simulink model "N3Z_tonetest (conflicted)"  (R2014b)
settings: Solver=ode3  SolverMode=SingleTasking  StartTime=0.0  StopTime=1e-4  FixedStep=fpgaclk  RelTol=1e-3
PreLoadFcn:
  | %fpgaclk=1/32.768e6
  | fpgaclk=1/49.162e6
  | 
  | SerialData=[1,zeros(1,11),1,0,0,1]
  | load ../N3workingG/window
  | win=win';  %Go back to using flatter and wider windowed sync function
  | %load ../N3workingG/hanning    %use Hahn window
  | 
  | load ../N3workingG/PREemphasis   %For pre-empasis and deemphasis FIRs
  | 
  | %LUT3=xls2LUT2('../IQI_Qdemod.xls'); LUT3
  | load ../N3workingG/LUT3
  | load ../N3workingG/FIRiq2
  | % xls2LUT
  | 
  | GetProgFiles
  | 
  | PinAssignments    %Get Pin references for TE0722
  | 
  | 
  | 
  | 
  | 
  | %LCD
  | LCDdata=[LCD_D7,LCD_D6,LCD_D5,LCD_D4,LCD_D3,LCD_D2,LCD_D1,LCD_D0] %Note MSB...LSB!
  | LCDctrl=[LCD_E,LCD_RW,LCD_RS];
  | 
  | %for RS232 on pins 3 and 5 of USBB
  | 
  | %BT chip connections for WT12
  | 
  | RX_BT=RXD
  | TX_BT=TXD
  | 
  | RST_BB=RES
  | 
  | %PCMC=PCMC
  | %PCMS=PCMS
  | %PCMI=PCMI
  | %PCMO=PCMO
  | 
  | %Aliases:
  | SRDBT=PCMI
  | STDBT=PCMO
  | SCLK_BT=PCMC
  | SFS_BT=PCMS
  | 
  | %ADC control
  | 
  | %SDOA=SDOA
  | %SDOB=SDOB
  | %SCK=SCK
  | CONV=Csbar
  | CAL=Cal
  | 
  | ADC_G=[ADC_G3,ADC_G2,ADC_G1,ADC_G0]
  | %PD settings hard coded now
  | 
  | %%%%%%
  | TX_LOW=TX_Low
  | ... (+11 lines)
StartFcn:
  | SerialData=[1,zeros(1,11),1,0,0,1]
values from neighbouring files (symbols this model uses):
  ADC_G0 = {'P10'}    [PinAssignments.m]
  ADC_G1 = {'P11'}    [PinAssignments.m]
  ADC_G2 = {'N14'}    [PinAssignments.m]
  ADC_G3 = {'M11'}    [PinAssignments.m]
  Cal = {'L12'}    [PinAssignments.m]
  Csbar = {'M12'}    [PinAssignments.m]
  LCD_D0 = {'J13'}    [PinAssignments.m]
  LCD_D1 = {'J14'}    [PinAssignments.m]
  LCD_D2 = {'F15'}    [PinAssignments.m]
  LCD_D3 = {'H14'}    [PinAssignments.m]
  LCD_D4 = {'G12'}    [PinAssignments.m]
  LCD_D5 = {'L15'}    [PinAssignments.m]
  LCD_D6 = {'M14'}    [PinAssignments.m]
  LCD_D7 = {'K15'}    [PinAssignments.m]
  PCMC = {'H11'}    [PinAssignments.m]
  PCMI = {'H12'}    [PinAssignments.m]
  PCMO = {'N13'}    [PinAssignments.m]
  PCMS = {'M10'}    [PinAssignments.m]
  RES = {'G11'}    [PinAssignments.m]
  RXD = {'H13'}    [PinAssignments.m]
  TX_Low = {'P15'}    [PinAssignments.m]
  TXD = {'P13'}    [PinAssignments.m]
undefined symbols (not defined in the file or in its folder): AXI4, FIRRX, FIRTX, Lite
libraries: xbsIndex_r4 x1251, MyFunctions x43
(part 3 of 9)

== system N3Z_tonetest (conflicted)/LevelMonitor ==
  note: Add 13-1 (make quicker and reduce level to 7 bits -2014) bits above and below to get ~1.25s time constant
  note: Top 2 bits are sign extended!
  note: Feb 2011 added 1 bit to AddSub unit March 2014, removed 2 bits!
  note: Add lower oscillating bit (but now gives twice the value) - shorter integration
      | but take slice 2 bits lower down - also saturate so as not to wrap around!
  In1 : Inport
  En : Inport  Port=2
  RstPeak : Inport  Port=3
  AddSub : xbsIndex_r4/AddSub  mode=Addition or Subtraction  use_carryin=off  use_carryout=off  en=off  latency=0  precision=User Defined  arith_type=Unsigned  n_bits=22-8+14-1-1  bin_pt=0  quantization=Truncate  overflow=Saturate  use_behavioral_HDL=off  hw_selection=Fabric  pipelined=off  dbl_ovrd=off  block_type=addsub
      settings: block_version=12.2
  AddSub1 : xbsIndex_r4/AddSub  mode=Addition or Subtraction  use_carryin=off  use_carryout=off  en=off  latency=0  precision=User Defined  arith_type=Unsigned  n_bits=8  bin_pt=0  quantization=Truncate  overflow=Saturate  use_behavioral_HDL=off  hw_selection=Fabric  pipelined=off  dbl_ovrd=off  block_type=addsub
      settings: block_version=12.2
  Concat : xbsIndex_r4/Concat  num_inputs=2  dbl_ovrd=off  block_type=concat
      settings: block_version=12.2
  Constant : xbsIndex_r4/Constant  const=0  gui_display_data_type=Fixed-point  arith_type=Signed (2's comp)  n_bits=8  bin_pt=0  preci_type=Single  exp_width=8  frac_width=24  explicit_period=on  period=fpgaclk  equ=P=C  opselect=C  inp2=PCIN>>17  opr=+  inp1=P  carry=CIN  dbl_ovrd=off  block_type=constant
  Convert : xbsIndex_r4/Convert  gui_display_data_type=Boolean  arith_type=Boolean  n_bits=16  bin_pt=14  float_type=Single  exp_bits=8  fraction_bits=24  quantization=Truncate  overflow=Wrap  en=off  latency=0  pipeline=off  dbl_ovrd=off  block_type=convert
      settings: block_version=12.2
  Convert1 : xbsIndex_r4/Convert  gui_display_data_type=Fixed-point  arith_type=Boolean  n_bits=16  bin_pt=14  float_type=Single  exp_bits=8  fraction_bits=24  quantization=Truncate  overflow=Wrap  en=off  latency=0  pipeline=off  dbl_ovrd=off  block_type=convert
      settings: block_version=12.2
  Convert2 : xbsIndex_r4/Convert  gui_display_data_type=Fixed-point  arith_type="Signed  (2's comp)"  n_bits=8  bin_pt=0  float_type=Single  exp_bits=8  fraction_bits=24  quantization=Truncate  overflow=Wrap  en=off  latency=0  pipeline=off  dbl_ovrd=off  block_type=convert
      settings: block_version=12.2
  Counter : xbsIndex_r4/Counter  cnt_type=Free Running  cnt_to=Inf  operation=Up  start_count=0  cnt_by_val=1  arith_type=Unsigned  n_bits=8+13-1  bin_pt=0  load_pin=off  rst=off  en=on  explicit_period=on  period=fpgaclk  use_behavioral_HDL=off  implementation=Fabric  dbl_ovrd=off  block_type=counter
      settings: block_version=12.2
  Counter1 : xbsIndex_r4/Counter  cnt_type=Free Running  cnt_to=Inf  operation=Up  start_count=0  cnt_by_val=1  arith_type=Unsigned  n_bits=1  bin_pt=0  load_pin=off  rst=off  en=on  explicit_period=on  period=fpgaclk  use_behavioral_HDL=off  implementation=Fabric  dbl_ovrd=off  block_type=counter
      settings: block_version=12.2
  Monostable : MyFunctions/Monostable
  Monostable1 : MyFunctions/Monostable
  Register : xbsIndex_r4/Register  init=0  rst=on  en=on  dbl_ovrd=off  block_type=register
      settings: block_version=12.2
  Register1 : xbsIndex_r4/Register  init=0  rst=off  en=on  dbl_ovrd=off  block_type=register
      settings: block_version=12.2
  Register2 : xbsIndex_r4/Register  init=0  rst=on  en=on  dbl_ovrd=off  block_type=register
  Register3 : xbsIndex_r4/Register  init=0  rst=off  en=on  dbl_ovrd=off  block_type=register
      settings: block_version=12.2
  Relational : xbsIndex_r4/Relational  mode=a<b  op_type=Bool  en=off  latency=1  dbl_ovrd=off  block_type=relational
  Slice1 : xbsIndex_r4/Slice  nbits=1  boolean_output=off  mode=Upper Bit Location + Width  bit1=0  base1=MSB of Input  bit0=0  base0=LSB of Input  dbl_ovrd=off  block_type=slice
      settings: block_version=12.2
  Slice2 : xbsIndex_r4/Slice  nbits=1  boolean_output=off  mode=Upper Bit Location + Width  bit1=0  base1=MSB of Input  bit0=0  base0=LSB of Input  dbl_ovrd=off  block_type=slice
      settings: block_version=12.2
  Slice3 : xbsIndex_r4/Slice  nbits=7  boolean_output=off  mode=Upper Bit Location + Width  bit1=0  base1=MSB of Input  bit0=0  base0=LSB of Input  dbl_ovrd=off  block_type=slice
      settings: block_version=12.2
  Slice4 : xbsIndex_r4/Slice  nbits=8  boolean_output=off  mode=Upper Bit Location + Width  bit1=-2  base1=MSB of Input  bit0=0  base0=LSB of Input  dbl_ovrd=off  block_type=slice
      settings: block_version=12.2
  SignalLevel : Outport
  PkSignal : Outport  Port=2
  wires:
  In1/1 -> Slice1/1, Slice4/1
  AddSub/1 -> Register/1
  En/1 -> Register3/2, Register/3, Counter/1
  Slice1/1 -> Convert/1
  Convert/1 -> AddSub1/3, AddSub/3
  Register/1 -> Slice3/1, AddSub/1
  Counter/1 -> Slice2/1
  Monostable/1 -> Convert1/1
  Convert1/1 -> Register/2, Register1/2, Counter1/1
  Slice2/1 -> Monostable/1
  Slice3/1 -> Register1/1
  Slice4/1 -> Convert2/1
  Convert2/1 -> AddSub/2, AddSub1/2
  Register1/1 -> Concat/1
  Counter1/1 -> Concat/2
  Concat/1 -> SignalLevel/1
  Constant/1 -> AddSub1/1
  Register2/1 -> PkSignal/1, Relational/1
  AddSub1/1 -> Register3/1
  Register3/1 -> Relational/2, Register2/1
  Relational/1 -> Monostable1/1
  Monostable1/1 -> Register2/3
  RstPeak/1 -> Register2/2

== system N3Z_tonetest (conflicted)/LevelMonitor1 ==
  In1 : Inport
  En : Inport  Port=2
  RstPeak : Inport  Port=3
  AddSub1 : xbsIndex_r4/AddSub  mode=Addition or Subtraction  use_carryin=off  use_carryout=off  en=off  latency=0  precision=User Defined  arith_type=Unsigned  n_bits=8  bin_pt=0  quantization=Truncate  overflow=Saturate  use_behavioral_HDL=off  hw_selection=Fabric  pipelined=off  dbl_ovrd=off  block_type=addsub
      settings: block_version=12.2
  Constant : xbsIndex_r4/Constant  const=0  gui_display_data_type=Fixed-point  arith_type=Signed (2's comp)  n_bits=8  bin_pt=0  preci_type=Single  exp_width=8  frac_width=24  explicit_period=on  period=fpgaclk  equ=P=C  opselect=C  inp2=PCIN>>17  opr=+  inp1=P  carry=CIN  dbl_ovrd=off  block_type=constant
  Convert : xbsIndex_r4/Convert  gui_display_data_type=Boolean  arith_type=Boolean  n_bits=16  bin_pt=14  float_type=Single  exp_bits=8  fraction_bits=24  quantization=Truncate  overflow=Wrap  en=off  latency=0  pipeline=off  dbl_ovrd=off  block_type=convert
      settings: block_version=12.2
  Convert2 : xbsIndex_r4/Convert  gui_display_data_type=Fixed-point  arith_type="Signed  (2's comp)"  n_bits=8  bin_pt=0  float_type=Single  exp_bits=8  fraction_bits=24  quantization=Truncate  overflow=Wrap  en=off  latency=0  pipeline=off  dbl_ovrd=off  block_type=convert
      settings: block_version=12.2
  Monostable1 : MyFunctions/Monostable
  Register2 : xbsIndex_r4/Register  init=0  rst=on  en=on  dbl_ovrd=off  block_type=register
  Register3 : xbsIndex_r4/Register  init=0  rst=off  en=on  dbl_ovrd=off  block_type=register
      settings: block_version=12.2
  Relational : xbsIndex_r4/Relational  mode=a<b  op_type=Bool  en=off  latency=1  dbl_ovrd=off  block_type=relational
  Slice1 : xbsIndex_r4/Slice  nbits=1  boolean_output=off  mode=Upper Bit Location + Width  bit1=0  base1=MSB of Input  bit0=0  base0=LSB of Input  dbl_ovrd=off  block_type=slice
      settings: block_version=12.2
  Slice4 : xbsIndex_r4/Slice  nbits=8  boolean_output=off  mode=Upper Bit Location + Width  bit1=0  base1=MSB of Input  bit0=0  base0=LSB of Input  dbl_ovrd=off  block_type=slice
      settings: block_version=12.2
  PkSignal : Outport
  wires:
  In1/1 -> Slice1/1, Slice4/1
  En/1 -> Register3/2
  Slice1/1 -> Convert/1
  Convert/1 -> AddSub1/3
  Slice4/1 -> Convert2/1
  Convert2/1 -> AddSub1/2
  Constant/1 -> AddSub1/1
  Register2/1 -> Relational/1, PkSignal/1
  AddSub1/1 -> Register3/1
  Register3/1 -> Register2/1, Relational/2
  Relational/1 -> Monostable1/1
  Monostable1/1 -> Register2/3
  RstPeak/1 -> Register2/2

== system N3Z_tonetest (conflicted)/LoranPulsedetect ==
  Signal : Inport
  Strobe : Inport  Port=2
  FastLevelMonitor : Subsystem
  LoranTrigger : Subsystem
  LranPass : Subsystem
  Trig : Outport
  wires:
  LranPass/1(Out1) -> FastLevelMonitor/1(In1), LoranTrigger/1(LoranSignal)
  FastLevelMonitor/1(SignalLevel) -> LoranTrigger/2(Thresh)
  Signal/1 -> LranPass/1(Signal)
  Strobe/1 -> LranPass/2(Strobe), FastLevelMonitor/2(En)
  LoranTrigger/1(Trig) -> Trig/1

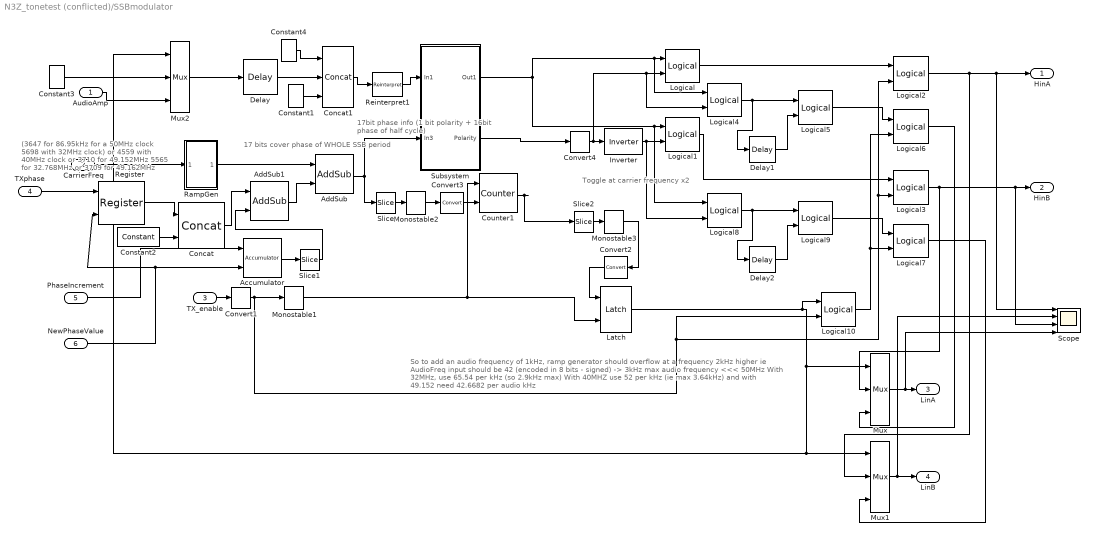
== system N3Z_tonetest (conflicted)/SSBmodulator  ==
  note: (3647 for 86.95kHz for a 50MHz clock
      | 5698 with 32MHz clock)
      | or 4559 with 40MHz clock
      | or 3710 for 49.152MHz
      | 5565 for 32.768MHz
      | or 3709 for 49.162MHz
  note: So to add an audio frequency of 1kHz, ramp generator should overflow at a frequency 2kHz higher
      | ie AudioFreq input should be 42 (encoded in 8 bits - signed) -> 3kHz max audio frequency <<< 50MHz
      | With 32MHz, use 65.54 per kHz (so 2.9kHz max)
      | With 40MHZ use 52 per kHz (ie max 3.64kHz)
      | and with 49.152 need 42.6682 per audio kHz
  note: Toggle at carrier frequency x2
  note: 17bit phase info
      | (1 bit polarity + 16bit phase of half cycle)
  note: 17 bits cover phase of WHOLE SSB period
  AudioAmp : Inport
  CarrierFreq : Inport  Port=2
  TX_enable : Inport  Port=3
  TXphase : Inport  Port=4
  PhaseIncrement : Inport  Port=5
  NewPhaseValue : Inport  Port=6
  Accumulator : xbsIndex_r4/Accumulator  operation=Add  n_bits=19  overflow=Wrap  scale=1  rst=on  hasbypass=off  infoeditControl=reset for floating point data type must be asserted for a minimum of 2 cycles  en=off  latency=0  msb_inp=100  msb=100  lsb=-100  use_behavioral_HDL=on  implementation=Fabric  dbl_ovrd=off  block_type=accum
      settings: block_version=VER_STRING_GOES_HERE
  AddSub : xbsIndex_r4/AddSub  mode=Addition  use_carryin=off  use_carryout=off  en=off  latency=1  precision=User Defined  arith_type=Unsigned  n_bits=17  bin_pt=0  quantization=Truncate  overflow=Wrap  use_behavioral_HDL=off  hw_selection=Fabric  pipelined=off  use_rpm=on  dbl_ovrd=off  block_type=addsub
      settings: block_version=VER_STRING_GOES_HERE
  AddSub1 : xbsIndex_r4/AddSub  mode=Addition  use_carryin=off  use_carryout=off  en=off  latency=0  precision=User Defined  arith_type=Unsigned  n_bits=17  bin_pt=0  quantization=Truncate  overflow=Wrap  use_behavioral_HDL=off  hw_selection=Fabric  pipelined=off  use_rpm=on  dbl_ovrd=off  block_type=addsub
      settings: block_version=VER_STRING_GOES_HERE
  Concat : xbsIndex_r4/Concat  num_inputs=2  dbl_ovrd=off  block_type=concat
      settings: block_version=12.2
  Concat1 : xbsIndex_r4/Concat  num_inputs=3  dbl_ovrd=off  block_type=concat
      settings: block_version=8.2.02
  Constant1 : xbsIndex_r4/Constant  const=0  gui_display_data_type=Fixed-point  arith_type=Unsigned  n_bits=7  bin_pt=0  preci_type=Single  exp_width=8  frac_width=24  explicit_period=on  period=fpgaclk  equ=P=C  opselect=C  inp2=PCIN>>17  opr=+  inp1=P  carry=CIN  dbl_ovrd=off  block_type=constant
      settings: block_version=VER_STRING_GOES_HERE
  Constant2 : xbsIndex_r4/Constant  const=0  gui_display_data_type=Fixed-point  arith_type=Unsigned  n_bits=1  bin_pt=0  preci_type=Single  exp_width=8  frac_width=24  explicit_period=on  period=fpgaclk  equ=P=C  opselect=C  inp2=PCIN>>17  opr=+  inp1=P  carry=CIN  dbl_ovrd=off  block_type=constant
      settings: block_version=12.2
  Constant3 : xbsIndex_r4/Constant  const=40  gui_display_data_type=Fixed-point  arith_type=Unsigned  n_bits=8  bin_pt=0  preci_type=Single  exp_width=8  frac_width=24  explicit_period=on  period=fpgaclk  equ=P=C  opselect=C  inp2=PCIN>>17  opr=+  inp1=P  carry=CIN  dbl_ovrd=off  block_type=constant
      settings: block_version=VER_STRING_GOES_HERE
  Constant4 : xbsIndex_r4/Constant  const=0  gui_display_data_type=Fixed-point  arith_type=Unsigned  n_bits=1  bin_pt=0  preci_type=Single  exp_width=8  frac_width=24  explicit_period=on  period=fpgaclk  equ=P=C  opselect=C  inp2=PCIN>>17  opr=+  inp1=P  carry=CIN  dbl_ovrd=off  block_type=constant
      settings: block_version=VER_STRING_GOES_HERE
  Convert{1..4} (4 alike) : xbsIndex_r4/Convert  gui_display_data_type=Fixed-point  arith_type=Boolean  n_bits=1  bin_pt=0  float_type=Single  exp_bits=8  fraction_bits=24  quantization=Truncate  overflow=Wrap  en=off  latency=0  pipeline=off  dbl_ovrd=off  block_type=convert
      settings: block_version=VER_STRING_GOES_HERE
  Counter1 : xbsIndex_r4/Counter  cnt_type=Free Running  cnt_to=Inf  operation=Up  start_count=0  cnt_by_val=1  arith_type=Unsigned  n_bits=7  bin_pt=0  load_pin=off  rst=on  en=on  explicit_period=off  period=1  use_behavioral_HDL=off  implementation=Fabric  use_rpm=off  dbl_ovrd=off  block_type=counter
      settings: block_version=VER_STRING_GOES_HERE
  Delay : xbsIndex_r4/Delay  rst=off  infoeditControl=Selection of Reset will increase slice count due to use of real FFs and instead of SRLs  en=off  latency=2  reg_retiming=off  dbl_ovrd=off  block_type=delay
      settings: infoedit=Hardware notes: A delay line is a chain, each link of which is an SRL16 followed by a flip-flop. If register retiming is enabled, the delay line is a chain of flip-flops.  block_version=VER_STRING_GOES_HERE
  Delay1 : xbsIndex_r4/Delay  rst=off  infoeditControl=Selection of Reset will increase slice count due to use of real FFs and instead of SRLs  en=off  latency=2  reg_retiming=off  dbl_ovrd=off  block_type=delay
      settings: block_version=12.2
  Delay2 : xbsIndex_r4/Delay  rst=off  infoeditControl=Selection of Reset will increase slice count due to use of real FFs and instead of SRLs  en=off  latency=2  reg_retiming=off  dbl_ovrd=off  block_type=delay
      settings: block_version=12.2
  Inverter : xbsIndex_r4/Inverter  en=off  latency=0  dbl_ovrd=off  block_type=inv
      settings: block_version=VER_STRING_GOES_HERE
  Latch : MyFunctions/Latch
      link override Register2: init=0  rst=on  en=on  dbl_ovrd=off
      link override Set1: arith_type=Boolean  const=1  n_bits=1  bin_pt=0  explicit_period=on  period=fpgaclk  equ=P=C  opselect=C  inp2=PCIN>>17  opr=+  inp1=P  carry=CIN  dbl_ovrd=off  gui_display_data_type=Boolean  preci_type=Single  exp_width=8  frac_width=24
  Logical : xbsIndex_r4/Logical  logical_function=AND  inputs=2  en=off  latency=2  precision=Full  arith_type=Unsigned  n_bits=16  bin_pt=0  align_bp=on  dbl_ovrd=off  block_type=logical
      settings: block_version=VER_STRING_GOES_HERE
  Logical1 : xbsIndex_r4/Logical  logical_function=AND  inputs=2  en=off  latency=2  precision=Full  arith_type=Unsigned  n_bits=16  bin_pt=0  align_bp=on  dbl_ovrd=off  block_type=logical
      settings: block_version=VER_STRING_GOES_HERE
  Logical{2..3,6..7,10} (5 alike) : xbsIndex_r4/Logical  logical_function=AND  inputs=2  en=off  latency=1  precision=Full  arith_type=Unsigned  n_bits=16  bin_pt=0  align_bp=on  dbl_ovrd=off  block_type=logical
      settings: block_version=VER_STRING_GOES_HERE
  Logical4 : xbsIndex_r4/Logical  logical_function=NAND  inputs=2  en=off  latency=1  precision=Full  arith_type=Unsigned  n_bits=16  bin_pt=0  align_bp=on  dbl_ovrd=off  block_type=logical
      settings: block_version=VER_STRING_GOES_HERE
  Logical5 : xbsIndex_r4/Logical  logical_function=AND  inputs=2  en=off  latency=0  precision=Full  arith_type=Unsigned  n_bits=16  bin_pt=0  align_bp=on  dbl_ovrd=off  block_type=logical
      settings: block_version=VER_STRING_GOES_HERE
  Logical8 : xbsIndex_r4/Logical  logical_function=NAND  inputs=2  en=off  latency=1  precision=Full  arith_type=Unsigned  n_bits=16  bin_pt=0  align_bp=on  dbl_ovrd=off  block_type=logical
      settings: block_version=VER_STRING_GOES_HERE
  Logical9 : xbsIndex_r4/Logical  logical_function=AND  inputs=2  en=off  latency=0  precision=Full  arith_type=Unsigned  n_bits=16  bin_pt=0  align_bp=on  dbl_ovrd=off  block_type=logical
      settings: block_version=VER_STRING_GOES_HERE
  Monostable1 : MyFunctions/Monostable
  Monostable2 : MyFunctions/Monostable
  Monostable3 : MyFunctions/Monostable
  Mux : xbsIndex_r4/Mux  inputs=2  en=off  latency=0  precision=Full  arith_type=Unsigned  n_bits=16  bin_pt=14  quantization=Truncate  overflow=Wrap  dbl_ovrd=off  block_type=mux
      settings: block_version=12.2
  Mux1 : xbsIndex_r4/Mux  inputs=2  en=off  latency=0  precision=Full  arith_type=Unsigned  n_bits=16  bin_pt=14  quantization=Truncate  overflow=Wrap  dbl_ovrd=off  block_type=mux
      settings: block_version=12.2
  Mux2 : xbsIndex_r4/Mux  inputs=2  en=off  latency=0  precision=Full  arith_type=Unsigned  n_bits=16  bin_pt=14  quantization=Truncate  overflow=Wrap  dbl_ovrd=off  block_type=mux
      settings: block_version=12.2
  RampGen : Subsystem
  Register : xbsIndex_r4/Register  init=0  rst=off  en=on  dbl_ovrd=off  block_type=register
      settings: block_version=12.2
  Reinterpret1 : xbsIndex_r4/Reinterpret  force_arith_type=on  arith_type=Unsigned  force_bin_pt=on  bin_pt=0  block_type=cast
      settings: infoedit="Changes signal type without altering the binary representation.   You can changed the signal between signed and unsigned, and relocate the binary point.<br><br>Hardware notes: In hardware this block costs nothing.<br><br>Example:  Suppose the input is 6 bits wide, signed, with 2 fractional bits, and the output is forced to unsigned with 0 fractional bits.  Then an input of -2.0 (1110.00 in binary 2's complement) becomes an output of 56 (111000 in binary)."  block_version=VER_STRING_GOES_HERE
  Scope : Scope  NumInputPorts=4
      settings: YMin=-5~-5~-5~-5  YMax=5~5~5~5  MaxDataPoints=50000
  Slice : xbsIndex_r4/Slice  nbits=1  boolean_output=off  mode=Upper Bit Location + Width  bit1=0  base1=MSB of Input  bit0=0  base0=LSB of Input  dbl_ovrd=off  block_type=slice
      settings: block_version=VER_STRING_GOES_HERE
  Slice1 : xbsIndex_r4/Slice  nbits=16  boolean_output=off  mode=Upper Bit Location + Width  bit1=0  base1=MSB of Input  bit0=0  base0=LSB of Input  dbl_ovrd=off  block_type=slice
      settings: block_version=VER_STRING_GOES_HERE
  Slice2 : xbsIndex_r4/Slice  nbits=1  boolean_output=off  mode=Upper Bit Location + Width  bit1=0  base1=MSB of Input  bit0=0  base0=LSB of Input  dbl_ovrd=off  block_type=slice
      settings: block_version=VER_STRING_GOES_HERE
  Subsystem : Subsystem
  HinA : Outport
  HinB : Outport  Port=2
  LinA : Outport  Port=3
  LinB : Outport  Port=4
  wires:
  Subsystem/1(Out1) -> Logical1/1, Logical8/1, Logical/1, Logical4/1
  Reinterpret1/1 -> Subsystem/1(In1)
  Counter1/1 -> Slice2/1
  Slice/1 -> Monostable2/1
  Monostable2/1 -> Convert3/1
  Convert4/1 -> Logical/2, Logical4/2, Inverter/1
  Inverter/1 -> Logical1/2, Logical8/2
  Delay/1 -> Concat1/2
  Concat1/1 -> Reinterpret1/1
  Constant4/1 -> Concat1/1
  Constant1/1 -> Concat1/3
  Logical/1 -> Logical2/1
  Logical1/1 -> Logical3/1
  TX_enable/1 -> Convert1/1
  Logical4/1 -> Logical5/1, Delay1/1
  Delay1/1 -> Logical5/2
  Logical8/1 -> Logical9/1, Delay2/1
  Delay2/1 -> Logical9/2
  Logical5/1 -> Logical6/1
  Logical9/1 -> Logical7/1
  Monostable1/1 -> Latch/2, Counter1/1
  Convert1/1 -> Monostable1/1, Logical10/2, Logical3/2, Logical2/2
  Slice2/1 -> Monostable3/1
  Latch/1 -> Mux/1, Mux1/1, Mux2/1, Logical10/1
  Monostable3/1 -> Convert2/1
  Logical2/1 -> Mux1/2, HinA/1, Scope/1
  Logical3/1 -> Mux/2, HinB/1, Scope/3
  Logical6/1 -> Mux/3
  Logical7/1 -> Mux1/3
  Logical10/1 -> Logical7/2, Logical6/2
  Mux/1 -> LinA/1, Scope/4
  Mux1/1 -> LinB/1, Scope/2
  Convert2/1 -> Latch/1
  Convert3/1 -> Counter1/2
  AudioAmp/1 -> Mux2/3
  Constant3/1 -> Mux2/2
  Mux2/1 -> Delay/1
  RampGen/1(Out1) -> AddSub/1
  AddSub/1 -> Subsystem/2(In3), Slice/1
  CarrierFreq/1 -> RampGen/1(In1)
  Constant2/1 -> Concat/2
  Subsystem/2(Polarity) -> Convert4/1
  Accumulator/1 -> Slice1/1
  Concat/1 -> AddSub1/1
  AddSub1/1 -> AddSub/2
  Slice1/1 -> AddSub1/2
  PhaseIncrement/1 -> Accumulator/1
  NewPhaseValue/1 -> Accumulator/2, Register/2
  TXphase/1 -> Register/1
  Register/1 -> Concat/1

== system N3Z_tonetest (conflicted)/Signed_Unsigned_offset ==
  In1 : Inport
  Concat : xbsIndex_r4/Concat  num_inputs=2  dbl_ovrd=off  block_type=concat
      settings: block_version=VER_STRING_GOES_HERE
  Inverter : xbsIndex_r4/Inverter  en=off  latency=0  dbl_ovrd=off  block_type=inv
      settings: xl_area=[0, 0, 0, 0, 0, 0, 0]  block_version=VER_STRING_GOES_HERE
  Slice2 : xbsIndex_r4/Slice  nbits=13  boolean_output=off  mode=Upper Bit Location + Width  bit1=-1  base1=MSB of Input  bit0=0  base0=LSB of Input  dbl_ovrd=off  block_type=slice
      settings: block_version=VER_STRING_GOES_HERE
  Slice3 : xbsIndex_r4/Slice  nbits=1  boolean_output=off  mode=Upper Bit Location + Width  bit1=0  base1=MSB of Input  bit0=0  base0=LSB of Input  dbl_ovrd=off  block_type=slice
      settings: block_version=VER_STRING_GOES_HERE
  Out1 : Outport
  wires:
  Slice2/1 -> Concat/2
  Slice3/1 -> Inverter/1
  Inverter/1 -> Concat/1
  In1/1 -> Slice2/1, Slice3/1
  Concat/1 -> Out1/1

== system N3Z_tonetest (conflicted)/Subsystem1 ==
  PCMin : Inport
  128kHz : Inport  Port=2
  SFS : Inport  Port=3
  Monostable2 : MyFunctions/Monostable
  Register2 : xbsIndex_r4/Register  init=0  rst=off  en=on  dbl_ovrd=off  block_type=register
      settings: block_version=10.1
  Subsystem1 : Subsystem
  AudioOut : Outport
  wires:
  Register2/1 -> Subsystem1/3(Conv)
  Monostable2/1 -> Register2/2
  PCMin/1 -> Subsystem1/1(SDOA)
  128kHz/1 -> Subsystem1/2(SCK), Monostable2/1
  SFS/1 -> Register2/1
  Subsystem1/1(ADCValueA) -> AudioOut/1

== system N3Z_tonetest (conflicted)/Subsystem2 ==
  note: Counts for 130us
  Signal : Inport
  Strbe : Inport  Port=2
  LoranPulseTrig : Inport  Port=3
  EnableGating : Inport  Port=4
  ADCvalue : xbsIndex_r4/Register  init=0  rst=off  en=on  dbl_ovrd=off  block_type=register
      settings: xl_area=[0, 0, 0, 0, 0, 0, 0]  block_version=VER_STRING_GOES_HERE
  Concat : xbsIndex_r4/Concat  num_inputs=2  dbl_ovrd=off  block_type=concat
      settings: block_version=12.2
  Constant : xbsIndex_r4/Constant  const=9  gui_display_data_type=Fixed-point  arith_type=Unsigned  n_bits=7  bin_pt=0  preci_type=Single  exp_width=8  frac_width=24  explicit_period=on  period=fpgaclk  equ=P=C  opselect=C  inp2=PCIN>>17  opr=+  inp1=P  carry=CIN  dbl_ovrd=off  block_type=constant
      settings: block_version=12.2
  Constant1 : xbsIndex_r4/Constant  const=55  gui_display_data_type=Fixed-point  arith_type=Unsigned  n_bits=7  bin_pt=0  preci_type=Single  exp_width=8  frac_width=24  explicit_period=on  period=fpgaclk  equ=P=C  opselect=C  inp2=PCIN>>17  opr=+  inp1=P  carry=CIN  dbl_ovrd=off  block_type=constant
      settings: block_version=12.2
  Constant2 : xbsIndex_r4/Constant  const=0  gui_display_data_type=Fixed-point  arith_type=Signed (2's comp)  n_bits=16  bin_pt=15  preci_type=Single  exp_width=8  frac_width=24  explicit_period=on  period=fpgaclk  equ=P=C  opselect=C  inp2=PCIN>>17  opr=+  inp1=P  carry=CIN  dbl_ovrd=off  block_type=constant
      settings: block_version=12.2
  Convert : xbsIndex_r4/Convert  gui_display_data_type=Fixed-point  arith_type=Unsigned  n_bits=1  bin_pt=0  float_type=Single  exp_bits=8  fraction_bits=24  quantization=Truncate  overflow=Wrap  en=off  latency=0  pipeline=off  dbl_ovrd=off  block_type=convert
      settings: block_version=12.2
  Convert1 : xbsIndex_r4/Convert  gui_display_data_type=Fixed-point  arith_type=Unsigned  n_bits=1  bin_pt=0  float_type=Single  exp_bits=8  fraction_bits=24  quantization=Truncate  overflow=Wrap  en=off  latency=0  pipeline=off  dbl_ovrd=off  block_type=convert
      settings: block_version=12.2
  Convert2 : xbsIndex_r4/Convert  gui_display_data_type=Fixed-point  arith_type=Boolean  n_bits=1  bin_pt=0  float_type=Single  exp_bits=8  fraction_bits=24  quantization=Truncate  overflow=Wrap  en=off  latency=0  pipeline=off  dbl_ovrd=off  block_type=convert
      settings: block_version=12.2
  Convert3 : xbsIndex_r4/Convert  gui_display_data_type=Fixed-point  arith_type=Boolean  n_bits=1  bin_pt=0  float_type=Single  exp_bits=8  fraction_bits=24  quantization=Truncate  overflow=Wrap  en=off  latency=0  pipeline=off  dbl_ovrd=off  block_type=convert
      settings: block_version=12.2
  Counter1 : xbsIndex_r4/Counter  cnt_type=Free Running  cnt_to=Inf  operation=Up  start_count=0  cnt_by_val=1  arith_type=Unsigned  n_bits=7  bin_pt=0  load_pin=off  rst=on  en=on  explicit_period=on  period=fpgaclk  use_behavioral_HDL=off  implementation=Fabric  dbl_ovrd=off  block_type=counter
      settings: block_version=12.2
  Delay : xbsIndex_r4/Delay  rst=off  infoeditControl=Selection of Reset will increase slice count due to use of real FFs and instead of SRLs  en=on  latency=15  reg_retiming=off  dbl_ovrd=off  block_type=delay
      settings: block_version=12.2
  Divide2 : Subsystem
  Inverter : xbsIndex_r4/Inverter  en=off  latency=0  dbl_ovrd=off  block_type=inv
      settings: block_version=12.2
  Latch : MyFunctions/Latch
      link override Set1: arith_type=Boolean  const=1  n_bits=1  bin_pt=0  explicit_period=on  period=fpgaclk  equ=P=C  opselect=C  inp2=PCIN>>17  opr=+  inp1=P  carry=CIN  dbl_ovrd=off  gui_display_data_type=Boolean  preci_type=Single  exp_width=8  frac_width=24
  Logical : xbsIndex_r4/Logical  logical_function=AND  inputs=2  en=off  latency=0  precision=Full  arith_type=Unsigned  n_bits=16  bin_pt=0  align_bp=on  dbl_ovrd=off  block_type=logical
      settings: block_version=12.2
  Logical1 : xbsIndex_r4/Logical  logical_function=AND  inputs=2  en=off  latency=0  precision=Full  arith_type=Unsigned  n_bits=16  bin_pt=0  align_bp=on  dbl_ovrd=off  block_type=logical
      settings: block_version=12.2
  Monostable : MyFunctions/Monostable
  Monostable1 : MyFunctions/Monostable
  Mux : xbsIndex_r4/Mux  inputs=4  en=off  latency=0  precision=Full  arith_type=Unsigned  n_bits=16  bin_pt=14  quantization=Truncate  overflow=Wrap  dbl_ovrd=off  block_type=mux
      settings: block_version=12.2
  Relational : xbsIndex_r4/Relational  mode=a>b  op_type=Bool  en=off  latency=1  dbl_ovrd=off  block_type=relational
      settings: block_version=12.2
  Relational1 : xbsIndex_r4/Relational  mode=a<=b  op_type=Bool  en=off  latency=1  dbl_ovrd=off  block_type=relational
      settings: block_version=12.2
  Slice : xbsIndex_r4/Slice  nbits=1  boolean_output=off  mode=Upper Bit Location + Width  bit1=0  base1=MSB of Input  bit0=0  base0=LSB of Input  dbl_ovrd=off  block_type=slice
      settings: block_version=12.2
  Archive : Outport
  CleanedUp : Outport  Port=2
  tag scope: LoranTrig=global
  wires:
  Delay/1 -> Archive/1, Mux/2, Divide2/1(In1)
  Signal/1 -> Delay/1
  Strbe/1 -> Delay/2, ADCvalue/2, Counter1/2
  ADCvalue/1 -> CleanedUp/1
  Monostable/1 -> Latch/1, [LoranTrig]
  Latch/1 -> Inverter/1, Convert/1
  Inverter/1 -> Counter1/1
  Counter1/1 -> Slice/1, Relational1/1, Relational/1
  Slice/1 -> Convert2/1
  Mux/1 -> ADCvalue/1
  Constant/1 -> Relational/2
  Constant1/1 -> Relational1/2
  Relational/1 -> Logical/1
  Relational1/1 -> Logical/2
  Logical/1 -> Convert1/1, Monostable1/1
  Convert/1 -> Concat/2
  Convert1/1 -> Concat/1
  Concat/1 -> Mux/1
  Constant2/1 -> Mux/5
  Divide2/1(Out1) -> Mux/3, Mux/4
  Convert2/1 -> Latch/2
  Logical1/1 -> Monostable/1
  LoranPulseTrig/1 -> Logical1/1
  EnableGating/1 -> Convert3/1
  Convert3/1 -> Logical1/2

== system N3Z_tonetest (conflicted)/Subsystem4 ==
  AudioIn : Inport
  Concat : xbsIndex_r4/Concat  num_inputs=2  dbl_ovrd=off  block_type=concat
      settings: block_version=9.2.01
  Convert1 : xbsIndex_r4/Convert  gui_display_data_type=Fixed-point  arith_type=Boolean  n_bits=16  bin_pt=14  float_type=Single  exp_bits=8  fraction_bits=24  quantization=Truncate  overflow=Wrap  en=off  latency=0  pipeline=off  dbl_ovrd=off  block_type=convert
      settings: block_version=9.2.01
  Convert2 : xbsIndex_r4/Convert  gui_display_data_type=Fixed-point  arith_type=Boolean  n_bits=16  bin_pt=14  float_type=Single  exp_bits=8  fraction_bits=24  quantization=Truncate  overflow=Wrap  en=off  latency=0  pipeline=off  dbl_ovrd=off  block_type=convert
      settings: block_version=9.2.01
  Monostable : MyFunctions/Monostable
  Monostable1 : MyFunctions/Monostable
  Mux : xbsIndex_r4/Mux  inputs=2  en=off  latency=0  precision=Full  arith_type=Unsigned  n_bits=16  bin_pt=14  quantization=Truncate  overflow=Wrap  dbl_ovrd=off  block_type=mux
      settings: block_version=9.2.01
  PCMclock : Subsystem
  Register : xbsIndex_r4/Register  init=0  rst=off  en=on  dbl_ovrd=off  block_type=register
      settings: block_version=10.1
  Register1 : xbsIndex_r4/Register  init=0  rst=off  en=on  dbl_ovrd=off  block_type=register
      settings: block_version=10.1
  Reinterpret : xbsIndex_r4/Reinterpret  force_arith_type=on  arith_type=Unsigned  force_bin_pt=on  bin_pt=0  block_type=reinterpret
      settings: block_version=9.2.01
  Slice : xbsIndex_r4/Slice  nbits=15  boolean_output=off  mode=Lower Bit Location + Width  bit1=0  base1=MSB of Input  bit0=0  base0=LSB of Input  dbl_ovrd=off  block_type=slice
      settings: infoedit="Extracts a given range of bits from each input sample and presents it at the output.  The output type is ordinarily unsigned with binary point at zero, but can be Boolean when the slice is one bit wide.<P><P>Hardware notes: In hardware this block costs nothing."  block_version=9.2.01
  Slice2 : xbsIndex_r4/Slice  nbits=1  boolean_output=off  mode=Upper Bit Location + Width  bit1=0  base1=MSB of Input  bit0=0  base0=LSB of Input  dbl_ovrd=off  block_type=slice
      settings: block_version=9.2.01
  PCMout : Outport
  128kHz : Outport  Port=2
  SFS : Outport  Port=3
  wires:
  PCMclock/2(Clk8kHz) -> Convert2/1
  Convert2/1 -> Monostable/1
  Concat/1 -> Mux/2
  Slice2/1 -> Concat/2, PCMout/1
  Slice/1 -> Concat/1
  Register1/1 -> Slice/1, Slice2/1
  Monostable1/1 -> Register1/2
  Mux/1 -> Register1/1
  Convert1/1 -> Monostable1/1, 128kHz/1
  PCMclock/1(128kHz) -> Convert1/1
  Register/1 -> Mux/3
  Monostable/1 -> Register/2, Mux/1
  AudioIn/1 -> Reinterpret/1
  PCMclock/3(STFS) -> SFS/1
  Reinterpret/1 -> Register/1

== system N3Z_tonetest (conflicted)/ToneDetect ==
  Assert4 : xbsIndex_r4/Assert  assert_type=off  type_source=Explicitly  gui_display_data_type=Fixed-point  arith_type="Signed  (2's comp)"  n_bits=16  bin_pt=14  preci_type=Single  exp_width=8  frac_width=24  assert_rate=on  rate_source=Explicitly  period=fpgaclk  output_port=on  block_type=assert
  Concat : xbsIndex_r4/Concat  num_inputs=4  dbl_ovrd=off  block_type=concat
      settings: block_version=9.2.01
  Constant1 : xbsIndex_r4/Constant  const=0  gui_display_data_type=Fixed-point  arith_type=Unsigned  n_bits=5  bin_pt=0  preci_type=Single  exp_width=8  frac_width=24  explicit_period=on  period=fpgaclk  equ=P=C  opselect=C  inp2=PCIN>>17  opr=+  inp1=P  carry=CIN  dbl_ovrd=off  block_type=constant
  Constant2 : xbsIndex_r4/Constant  const=0  gui_display_data_type=Fixed-point  arith_type=Unsigned  n_bits=8  bin_pt=0  preci_type=Single  exp_width=8  frac_width=24  explicit_period=on  period=fpgaclk  equ=P=C  opselect=C  inp2=PCIN>>17  opr=+  inp1=P  carry=CIN  dbl_ovrd=off  block_type=constant
  Constant4 : xbsIndex_r4/Constant  const=0  gui_display_data_type=Boolean  arith_type=Boolean  n_bits=1  bin_pt=0  preci_type=Single  exp_width=8  frac_width=24  explicit_period=on  period=fpgaclk  equ=P=C  opselect=C  inp2=PCIN>>17  opr=+  inp1=P  carry=CIN  dbl_ovrd=off  block_type=constant
      settings: block_version=VER_STRING_GOES_HERE
  Convert1 : xbsIndex_r4/Convert  gui_display_data_type=Fixed-point  arith_type=Boolean  n_bits=16  bin_pt=0  float_type=Single  exp_bits=8  fraction_bits=24  quantization=Truncate  overflow=Wrap  en=off  latency=0  pipeline=off  dbl_ovrd=off  block_type=convert
      settings: xl_area=[0 0 0 0 0 0 0]  block_version=VER_STRING_GOES_HERE
  Convert3 : xbsIndex_r4/Convert  gui_display_data_type=Fixed-point  arith_type=Boolean  n_bits=16  bin_pt=0  float_type=Single  exp_bits=8  fraction_bits=24  quantization=Truncate  overflow=Wrap  en=off  latency=0  pipeline=off  dbl_ovrd=off  block_type=convert
      settings: xl_area=[0 0 0 0 0 0 0]  block_version=VER_STRING_GOES_HERE
  Delay : xbsIndex_r4/Delay  rst=off  infoeditControl=Selection of Reset will increase slice count due to use of real FFs and instead of SRLs  en=off  latency=5  reg_retiming=off  dbl_ovrd=off  block_type=delay
      settings: infoedit=Hardware notes: A delay line is a chain, each link of which is an SRL16 or SRL32 followed by a flip-flop.
  Mult : xbsIndex_r4/Mult  precision=Full  arith_type="Signed  (2's comp)"  n_bits=16  bin_pt=14  quantization=Truncate  overflow=Wrap  en=off  latency=3  use_behavioral_HDL=off  opt=Speed  use_embedded=on  optimum_pipeline=off  pipeline=on  dbl_ovrd=off  use_rpm=on  placement_style=Triangular  block_type=mult
  Mux : xbsIndex_r4/Mux  inputs=8  en=off  latency=1  precision=Full  arith_type=Unsigned  n_bits=16  bin_pt=14  quantization=Truncate  overflow=Wrap  dbl_ovrd=off  block_type=mux
      settings: xl_area=[16 0 0 32 0 0 0]  block_version=VER_STRING_GOES_HERE
  OutputRegister : Subsystem
  PicoBlaze6 : xbsIndex_r4/Black Box  init_code=kcpsm6_CE_256_4k_config  sim_method=Inactive  verbose=off  block_type=blackbox2
  ROM : xbsIndex_r4/ROM  depth=256  initVector=(2^15-1)*sin(pi*(0:255)/128)  distributed_mem=Block RAM  rst=off  init_reg=0  en=off  latency=1  gui_display_data_type=Fixed-point  arith_type="Signed  (2's comp)"  n_bits=16  bin_pt=0  preci_type=Single  exp_width=8  frac_width=24  optimize=Area  use_rpm=on  dbl_ovrd=off  block_type=sprom
  Register : xbsIndex_r4/Register  init=0  rst=off  en=on  dbl_ovrd=off  block_type=register
  Slice : xbsIndex_r4/Slice  nbits=8  boolean_output=off  mode=Lower Bit Location + Width  bit1=0  base1=MSB of Input  bit0=0  base0=LSB of Input  dbl_ovrd=off  block_type=slice
      settings: block_version=8.2.02
  Slice1 : xbsIndex_r4/Slice  nbits=8  boolean_output=off  mode=Lower Bit Location + Width  bit1=0  base1=MSB of Input  bit0=8  base0=LSB of Input  dbl_ovrd=off  block_type=slice
      settings: block_version=8.2.02
  Slice2 : xbsIndex_r4/Slice  nbits=3  boolean_output=off  mode=Lower Bit Location + Width  bit1=0  base1=MSB of Input  bit0=0  base0=LSB of Input  dbl_ovrd=off  block_type=slice
      settings: block_version=VER_STRING_GOES_HERE
  Slice3 : xbsIndex_r4/Slice  nbits=8  boolean_output=off  mode=Upper Bit Location + Width  bit1=-8  base1=MSB of Input  bit0=0  base0=LSB of Input  dbl_ovrd=off  block_type=slice
      settings: block_version=8.2.02
  Slice4 : xbsIndex_r4/Slice  nbits=8  boolean_output=off  mode=Upper Bit Location + Width  bit1=0  base1=MSB of Input  bit0=8  base0=LSB of Input  dbl_ovrd=off  block_type=slice
      settings: block_version=8.2.02
  Slice5 : xbsIndex_r4/Slice  nbits=1  boolean_output=off  mode=Lower Bit Location + Width  bit1=0  base1=MSB of Input  bit0=0  base0=LSB of Input  dbl_ovrd=off  block_type=slice
      settings: block_version=VER_STRING_GOES_HERE
  Slice9 : xbsIndex_r4/Slice  nbits=11  boolean_output=off  mode=Lower Bit Location + Width  bit1=0  base1=MSB of Input  bit0=0  base0=LSB of Input  dbl_ovrd=off  block_type=slice
      settings: block_version=VER_STRING_GOES_HERE
  TDPicoAddress : xbsIndex_r4/Gateway Out  inherit_from_input=off  hdl_port=on  rows=1  columns=1  UseAsDAC=off  DACChannel='1'  interface=None  automatic_assignment=on  address_offset=hex2dec('00')  intf_name=''  intf_description=''  timing_constraint=None  locs_specified=off  LOCs={}  io_standard={}  block_type=gatewayout
  TDPicoInstruction : xbsIndex_r4/Gateway In  gui_display_data_type=Fixed-point  arith_type=Unsigned  n_bits=18  bin_pt=0  preci_type=Single  exp_width=8  frac_width=24  rows=1  columns=1  quantization="Round  (unbiased: +/- Inf)"  overflow=Saturate  period=fpgaclk  UseAsADC=off  ADCChannel='1'  interface=None  automatic_assignment=on  address_offset=hex2dec('00')  intf_name=''  intf_description=''  default_value=0  timing_constraint=None  locs_specified=off  LOCs={}  io_standard={}  inherit_from_input=off  hdl_port=on  dbl_ovrd=off  block_type=gatewayin
  TD_portID : xbsIndex_r4/Gateway Out  inherit_from_input=off  hdl_port=on  rows=1  columns=1  UseAsDAC=off  DACChannel='1'  interface=None  automatic_assignment=on  address_offset=hex2dec('00')  intf_name=''  intf_description=''  timing_constraint=None  locs_specified=off  LOCs={}  io_standard={'LVCMOS33'}  block_type=gatewayout
      settings: block_version=VER_STRING_GOES_HERE
  tag scope: NewTDcmd2user=global, SpeakerOn=global, StartToneAmp=global, TDcmd2user=global
  wires:
  PicoBlaze6/4 -> Slice2/1, OutputRegister/2(PortId), TD_portID/1
  PicoBlaze6/3 -> OutputRegister/1(Data)
  Mux/1 -> PicoBlaze6/2
  Constant4/1 -> Convert1/1
  Slice2/1 -> Assert4/1
  Convert1/1 -> PicoBlaze6/3, PicoBlaze6/4
  OutputRegister/1(Cmd2User) -> [TDcmd2user]
  OutputRegister/2(NewCmd) -> [NewTDcmd2user]
  Convert3/1 -> OutputRegister/3(Write)
  Assert4/1 -> Mux/1
  PicoBlaze6/1 -> Slice9/1
  PicoBlaze6/5 -> Convert3/1
  Slice/1 -> Mux/3
  Slice1/1 -> Mux/2
  [FilterredSignal] -> Slice/1, Slice1/1
  Constant1/1 -> Concat/1
  [Strobe] -> Concat/4
  Concat/1 -> Mux/4
  Slice3/1 -> Mux/6
  Slice4/1 -> Mux/5
  Constant2/1 -> Mux/9, Mux/7, Mux/8
  OutputRegister/3(LOMSB) -> ROM/1
  Mult/1 -> Register/1
  Register/1 -> Slice3/1, Slice4/1  "PrevousDemodValue"
  OutputRegister/4(DoDemod) -> Delay/1
  Slice9/1 -> TDPicoAddress/1
  TDPicoInstruction/1 -> PicoBlaze6/1
  [RstPicos] -> PicoBlaze6/5
  Delay/1 -> Register/2
  [FilterredSignal] -> Mult/1
  ROM/1 -> Mult/2
  OutputRegister/6(State) -> Slice5/1
  Slice5/1 -> [SpeakerOn]
  [TX_High] -> Concat/3
  OutputRegister/5(StartToneAmp) -> [StartToneAmp]
  [ToneDetectOff] -> Concat/2

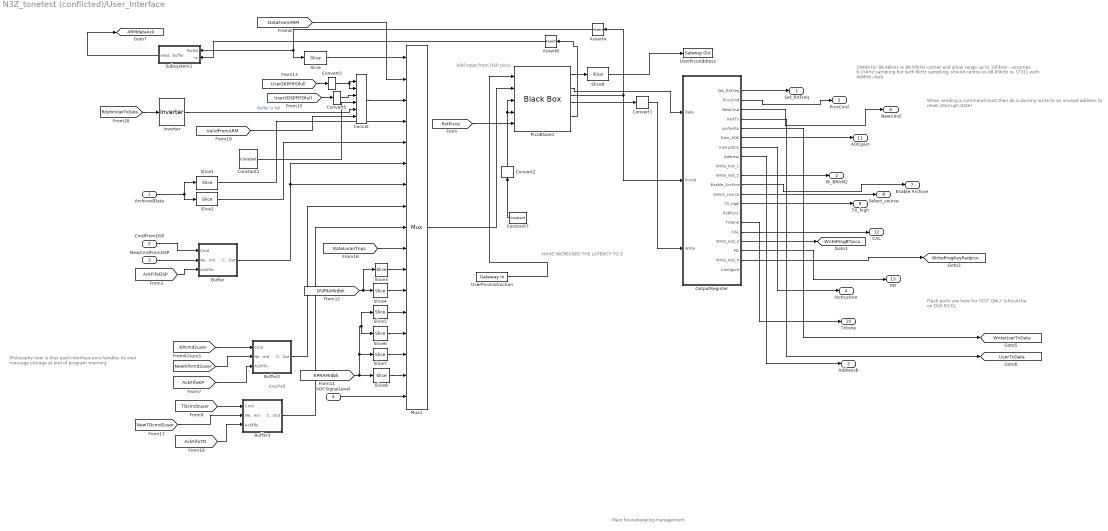
== system N3Z_tonetest (conflicted)/User_Interface ==
  note: When sending a command must then do a dummy write to an unused address
      | to reset interrupt state!
  note: 29689 for 88.48kHz
      |  ie 86.95kHz carrier and allow range up to 195kHz - assumes 6.15kHz sampling
      | but with 8kHz sampling, should centre on 88.95kHz ie 37311 with 40MHz clock
  note: Add input from DSP pico!
  note: Philosophy now is that each interface pico handles its own
      | message storage at end of program memory
  note: Main housekeeping management
  note: KeyPad
  note: Flash ports are here for TEST ONLY (should
      | be on DSP PICO)
  note: HAVE INCREASED THE LATENCY TO 2
  ArchivedData : Inport
  CmdFromDSP : Inport  Port=2
  NewCmdFromDSP : Inport  Port=3
  ADCSignalLevel : Inport  Port=4
  Assert4 : xbsIndex_r4/Assert  assert_type=off  type_source=Explicitly  gui_display_data_type=Fixed-point  arith_type="Signed  (2's comp)"  n_bits=16  bin_pt=14  preci_type=Single  exp_width=8  frac_width=24  assert_rate=on  rate_source=Explicitly  period=fpgaclk  output_port=on  block_type=assert
  Assert6 : xbsIndex_r4/Assert  assert_type=off  type_source=Explicitly  gui_display_data_type=Fixed-point  arith_type="Signed  (2's comp)"  n_bits=16  bin_pt=14  preci_type=Single  exp_width=8  frac_width=24  assert_rate=on  rate_source=Explicitly  period=fpgaclk  output_port=on  block_type=assert
  Buffer : Subsystem
  Buffer2 : Subsystem
  Buffer3 : Subsystem
  Concat : xbsIndex_r4/Concat  num_inputs=6  dbl_ovrd=off  block_type=concat
      settings: block_version=VER_STRING_GOES_HERE
  Constant1 : xbsIndex_r4/Constant  const=0  gui_display_data_type=Fixed-point  arith_type=Unsigned  n_bits=3  bin_pt=0  preci_type=Single  exp_width=8  frac_width=24  explicit_period=on  period=fpgaclk  equ=P=C  opselect=C  inp2=PCIN>>17  opr=+  inp1=P  carry=CIN  dbl_ovrd=off  block_type=constant
      settings: block_version=VER_STRING_GOES_HERE
  Constant7 : xbsIndex_r4/Constant  const=0  gui_display_data_type=Boolean  arith_type=Boolean  n_bits=1  bin_pt=0  preci_type=Single  exp_width=8  frac_width=24  explicit_period=on  period=fpgaclk  equ=P=C  opselect=C  inp2=PCIN>>17  opr=+  inp1=P  carry=CIN  dbl_ovrd=off  block_type=constant
      settings: block_version=VER_STRING_GOES_HERE
  Convert1 : xbsIndex_r4/Convert  gui_display_data_type=Fixed-point  arith_type=Boolean  n_bits=16  bin_pt=0  float_type=Single  exp_bits=8  fraction_bits=24  quantization=Truncate  overflow=Wrap  en=off  latency=0  pipeline=off  dbl_ovrd=off  block_type=convert
      settings: xl_area=[0 0 0 0 0 0 0]  block_version=VER_STRING_GOES_HERE
  Convert2 : xbsIndex_r4/Convert  gui_display_data_type=Fixed-point  arith_type=Boolean  n_bits=16  bin_pt=0  float_type=Single  exp_bits=8  fraction_bits=24  quantization=Truncate  overflow=Wrap  en=off  latency=0  pipeline=off  dbl_ovrd=off  block_type=convert
      settings: xl_area=[0, 0, 0, 0, 0, 0, 0]  block_version=VER_STRING_GOES_HERE
  Convert3 : xbsIndex_r4/Convert  gui_display_data_type=Fixed-point  arith_type=Unsigned  n_bits=1  bin_pt=0  float_type=Single  exp_bits=8  fraction_bits=24  quantization=Truncate  overflow=Wrap  en=off  latency=0  pipeline=off  dbl_ovrd=off  block_type=convert
      settings: xl_area=[0, 0, 0, 0, 0, 0, 0]  block_version=VER_STRING_GOES_HERE
  Convert5 : xbsIndex_r4/Convert  gui_display_data_type=Fixed-point  arith_type=Unsigned  n_bits=1  bin_pt=0  float_type=Single  exp_bits=8  fraction_bits=24  quantization=Truncate  overflow=Wrap  en=off  latency=0  pipeline=off  dbl_ovrd=off  block_type=convert
      settings: xl_area=[0, 0, 0, 0, 0, 0, 0]  block_version=VER_STRING_GOES_HERE
  Inverter : xbsIndex_r4/Inverter  en=off  latency=1  dbl_ovrd=off  block_type=inv
  Mux1 : xbsIndex_r4/Mux  inputs=16  en=off  latency=1  precision=Full  arith_type=Unsigned  n_bits=16  bin_pt=14  quantization=Truncate  overflow=Wrap  dbl_ovrd=off  block_type=mux
      settings: block_version=12.2
  OutputRegister : Subsystem
  PicoBlaze1 : xbsIndex_r4/Black Box  init_code=kcpsm6_CE_256_4k_config  sim_method=Inactive  verbose=off  block_type=blackbox2
  Slice : xbsIndex_r4/Slice  nbits=4  boolean_output=off  mode=Lower Bit Location + Width  bit1=0  base1=MSB of Input  bit0=0  base0=LSB of Input  dbl_ovrd=off  block_type=slice
      settings: block_version=VER_STRING_GOES_HERE
  Slice{1,4,6,8} (4 alike) : xbsIndex_r4/Slice  nbits=8  boolean_output=off  mode=Lower Bit Location + Width  bit1=0  base1=MSB of Input  bit0=0  base0=LSB of Input  dbl_ovrd=off  block_type=slice
      settings: block_version=VER_STRING_GOES_HERE
  Slice{2..3,5,7} (4 alike) : xbsIndex_r4/Slice  nbits=8  boolean_output=off  mode=Lower Bit Location + Width  bit1=0  base1=MSB of Input  bit0=8  base0=LSB of Input  dbl_ovrd=off  block_type=slice
      settings: block_version=VER_STRING_GOES_HERE
  Slice9 : xbsIndex_r4/Slice  nbits=11  boolean_output=off  mode=Lower Bit Location + Width  bit1=0  base1=MSB of Input  bit0=0  base0=LSB of Input  dbl_ovrd=off  block_type=slice
      settings: block_version=VER_STRING_GOES_HERE
  Subsystem1 : Subsystem
  UserPicoAddress : xbsIndex_r4/Gateway Out  inherit_from_input=off  hdl_port=on  rows=1  columns=1  UseAsDAC=off  DACChannel='1'  interface=None  automatic_assignment=on  address_offset=hex2dec('00')  intf_name=''  intf_description=''  timing_constraint=None  locs_specified=off  LOCs={}  io_standard={}  block_type=gatewayout
  UserPicoInstruction : xbsIndex_r4/Gateway In  gui_display_data_type=Fixed-point  arith_type=Unsigned  n_bits=18  bin_pt=0  preci_type=Single  exp_width=8  frac_width=24  rows=1  columns=1  quantization="Round  (unbiased: +/- Inf)"  overflow=Saturate  period=fpgaclk  UseAsADC=off  ADCChannel='1'  interface=None  automatic_assignment=on  address_offset=hex2dec('00')  intf_name=''  intf_description=''  default_value=0  timing_constraint=None  locs_specified=off  LOCs={}  io_standard={}  inherit_from_input=off  hdl_port=on  dbl_ovrd=off  block_type=gatewayin
  Set_RXFreq : Outport
  W_BRAM2 : Outport  Port=2
  Addressb : Outport  Port=3
  Instruction : Outport  Port=4
  PicoCmd : Outport  Port=5
  NewCmd : Outport  Port=6
  Enable Archive : Outport  Port=7
  Select_source : Outport  Port=8
  TX_high : Outport  Port=9
  TXtone : Outport  Port=10
  ADCgain : Outport  Port=11
  CAL : Outport  Port=12
  PD : Outport  Port=13
  tag scope: ARMdataAck=global, UserTxData=global, WriteProgBTpico=global, WriteProgKeyPadpico=global, WriteUserTxData=global
  wires:
  Constant7/1 -> Convert2/1
  Concat/1 -> Mux1/3
  Subsystem1/1(read_buffer) -> [ARMdataAck]
  OutputRegister/5(uartwrite) -> [WriteUserTxData]
  OutputRegister/4(UartTx) -> [UserTxData]
  OutputRegister/6(Gain_ADC) -> ADCgain/1
  OutputRegister/7(Instruction) -> Instruction/1
  OutputRegister/8(Address) -> Addressb/1
  Slice/1 -> Mux1/1
  OutputRegister/1(Set_RXFreq) -> Set_RXFreq/1
  OutputRegister/10(Write_Inst_2) -> W_BRAM2/1
  OutputRegister/2(PicoCmd) -> PicoCmd/1
  ArchivedData/1 -> Slice1/1, Slice2/1
  Slice1/1 -> Mux1/4
  Slice2/1 -> Mux1/5
  OutputRegister/11(Enable_Archive) -> Enable Archive/1
  OutputRegister/12(Select_source) -> Select_source/1
  OutputRegister/13(TX_high) -> TX_high/1
  OutputRegister/3(NewCmd) -> NewCmd/1
  OutputRegister/15(TXtone) -> TXtone/1
  CmdFromDSP/1 -> Buffer/1(Cmd)
  NewCmdFromDSP/1 -> Buffer/2(NewCmd)
  PicoBlaze1/1 -> Slice9/1
  PicoBlaze1/4 -> Assert4/1, OutputRegister/2(PortId)
  PicoBlaze1/3 -> OutputRegister/1(Data)
  PicoBlaze1/5 -> Convert1/1
  PicoBlaze1/7 -> Assert6/1
  Convert1/1 -> OutputRegister/3(Write)
  OutputRegister/16(CAL) -> CAL/1
  OutputRegister/17(Write_Inst_3) -> [WriteProgBTpico]
  [AckFifoDSP] -> Buffer/3(AckFifo)
  [KPcmd2user] -> Buffer2/1(Cmd)
  [NewKPcmd2user] -> Buffer2/2(NewCmd)
  [AckFifoKP] -> Buffer2/3(AckFifo)
  OutputRegister/18(PD) -> PD/1
  Buffer/1(CmdOut) -> Mux1/7, Mux1/6
  Buffer2/1(CmdOut) -> Mux1/8
  [RdyforUserTxData] -> Inverter/1
  OutputRegister/19(Write_Inst_4) -> [WriteProgKeyPadpico]
  [DSPRAMrdbk] -> Slice3/1, Slice4/1
  [KPRAMrdbk] -> Slice6/1, Slice5/1, Slice7/1, Slice8/1
  [User2KPFIFOfull] -> Convert3/1
  [User2DSPFIFOfull] -> Convert5/1
  Slice3/1 -> Mux1/11
  Slice4/1 -> Mux1/12
  Slice5/1 -> Mux1/13
  Slice6/1 -> Mux1/14
  Slice7/1 -> Mux1/15
  Slice8/1 -> Mux1/16
  Mux1/1 -> PicoBlaze1/2
  ADCSignalLevel/1 -> Mux1/17
  Assert4/1 -> Slice/1, Subsystem1/1(PortId)
  Assert6/1 -> Subsystem1/2(rs)
  Constant1/1 -> Concat/4
  [RateLoranTrips] -> Mux1/10
  [TDcmd2user] -> Buffer3/1(Cmd)
  [NewTDcmd2user] -> Buffer3/2(NewCmd)
  [AckFifoTD] -> Buffer3/3(AckFifo)
  Buffer3/1(CmdOut) -> Mux1/9
  [ValidFromARM] -> Concat/6
  [DataFromARM] -> Mux1/2
  Convert3/1 -> Concat/1, Concat/2
  Convert5/1 -> Concat/3
  Inverter/1 -> Concat/5  "Buffer is full"
  Slice9/1 -> UserPicoAddress/1
  UserPicoInstruction/1 -> PicoBlaze1/1
  Convert2/1 -> PicoBlaze1/4, PicoBlaze1/3
  [RstPicos] -> PicoBlaze1/5
